simulink model "board_virgin_lab2"  (R2015a)
settings: Solver=ode3  StartTime=0.0  StopTime=inf  FixedStep=0.001  RelTol=1e-3
values from neighbouring files (symbols this model uses):
  T1gain = Pt1(1)    [callback.m]
  T1offset = Pt1(2)    [callback.m]
  T2gain = Pt2(1)    [callback.m]
  T2offset = Pt2(2)    [callback.m]
  Xgain = Px(1)    [callback.m]
  Xoffset = Px(2)    [callback.m]
  Ygain = Py(1)    [callback.m]
  Yoffset = Py(2)    [callback.m]
libraries: PoliArd x14, simulink x4
settings Model: ExtModeTrigDuration=2  Creator=User  LastModifiedBy=user
settings OptimizationCC: OptimizeModelRefInitCode=on  LifeSpan=1
settings DebuggingCC: UnderspecifiedInitializationDetection=Classic  MergeDetectMultiDrivingBlocksExec=none
settings HardwareCC: ProdLargestAtomicInteger=Long  ProdLargestAtomicFloat=Double  ProdEndianess=LittleEndian  ProdHWDeviceType=ARM Compatible->ARM Cortex
settings RTWCC: SystemTargetFile=realtime.tlc  GenerateMakefile=off  TemplateMakefile=realtime.tmf  Description=Run on Target Hardware  RTWVerbose=off
settings ERTTargetCC: CombineOutputUpdateFcns=off  ExtModeTransport=3  ExtModeMexFile=ext_serial_win32_comm_rtt  ExtModeMexArgs=0 1 9600  InlinedParameterPlacement=Hierarchical  ERTSrcFileBannerTemplate=realtime_code_template.cgt  ERTHdrFileBannerTemplate=realtime_code_template.cgt  ERTDataSrcFileTemplate=realtime_code_template.cgt  ERTDataHdrFileTemplate=realtime_code_template.cgt  ERTCustomFileTemplate=realtime_file_process.tlc

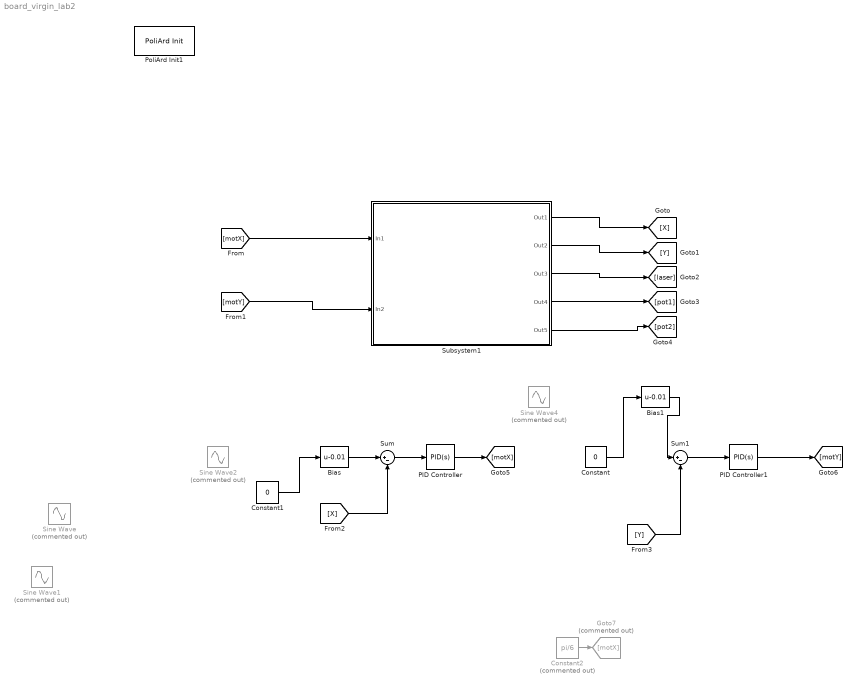
== system board_virgin_lab2 ==
  Bias : Bias  Bias=-0.01
  Bias1 : Bias  Bias=-0.01
  Constant : Constant  Value=0
  Constant1 : Constant  Value=0
  Constant2 : Constant  Commented=on  Value=pi/6
  Goto7 : Goto  Commented=on  GotoTag=motX
  PID Controller : simulink/Continuous/PID Controller  Controller=PID  TimeDomain=Continuous-time  SampleTime=-1  IntegratorMethod=Forward Euler  FilterMethod=Forward Euler  Form=Parallel  UseFilter=on  ControllerParametersSource=internal  P=3  I=1.5  D=2.5  N=5.45  InitialConditionSource=internal  InitialConditionForIntegrator=0  InitialConditionForFilter=0  ExternalReset=none  LimitOutput=off  UpperSaturationLimit=inf  LowerSaturationLimit=-inf  LinearizeAsGain=on  AntiWindupMode=none  Kb=1  TrackingMode=off  Kt=1  PParamMin=[]  PParamMax=[]  IParamMin=[]  IParamMax=[]  DParamMin=[]  DParamMax=[]  NParamMin=[]  NParamMax=[]  KbParamMin=[]  KbParamMax=[]  KtParamMin=[]  KtParamMax=[]  POutMin=[]  POutMax=[]  IOutMin=[]  IOutMax=[]  DOutMin=[]  DOutMax=[]  NOutMin=[]  NOutMax=[]  KbOutMin=[]  KbOutMax=[]  KtOutMin=[]  KtOutMax=[]  IntegratorOutMin=[]  IntegratorOutMax=[]  FilterOutMin=[]  FilterOutMax=[]  SumOutMin=[]  SumOutMax=[]  SumI1OutMin=[]  SumI1OutMax=[]  SumI2OutMin=[]  SumI2OutMax=[]  SumI3OutMin=[]  SumI3OutMax=[]  SumDOutMin=[]  SumDOutMax=[]  SaturationOutMin=[]  SaturationOutMax=[]  IntegratorContinuousStateAttributes=''  IntegratorStateMustResolveToSignalObject=off  IntegratorRTWStateStorageClass=Auto  FilterContinuousStateAttributes=''  FilterStateMustResolveToSignalObject=off  FilterRTWStateStorageClass=Auto  DifferentiatorICPrevScaledInput=0  DifferentiatorOutMin=[]  DifferentiatorOutMax=[]
  PID Controller1 : simulink/Continuous/PID Controller  Controller=PID  TimeDomain=Continuous-time  SampleTime=-1  IntegratorMethod=Forward Euler  FilterMethod=Forward Euler  Form=Parallel  UseFilter=on  ControllerParametersSource=internal  P=3  I=1.5  D=2.5  N=5.45  InitialConditionSource=internal  InitialConditionForIntegrator=0  InitialConditionForFilter=0  ExternalReset=none  LimitOutput=off  UpperSaturationLimit=inf  LowerSaturationLimit=-inf  LinearizeAsGain=on  AntiWindupMode=none  Kb=1  TrackingMode=off  Kt=1  PParamMin=[]  PParamMax=[]  IParamMin=[]  IParamMax=[]  DParamMin=[]  DParamMax=[]  NParamMin=[]  NParamMax=[]  KbParamMin=[]  KbParamMax=[]  KtParamMin=[]  KtParamMax=[]  POutMin=[]  POutMax=[]  IOutMin=[]  IOutMax=[]  DOutMin=[]  DOutMax=[]  NOutMin=[]  NOutMax=[]  KbOutMin=[]  KbOutMax=[]  KtOutMin=[]  KtOutMax=[]  IntegratorOutMin=[]  IntegratorOutMax=[]  FilterOutMin=[]  FilterOutMax=[]  SumOutMin=[]  SumOutMax=[]  SumI1OutMin=[]  SumI1OutMax=[]  SumI2OutMin=[]  SumI2OutMax=[]  SumI3OutMin=[]  SumI3OutMax=[]  SumDOutMin=[]  SumDOutMax=[]  SaturationOutMin=[]  SaturationOutMax=[]  IntegratorContinuousStateAttributes=''  IntegratorStateMustResolveToSignalObject=off  IntegratorRTWStateStorageClass=Auto  FilterContinuousStateAttributes=''  FilterStateMustResolveToSignalObject=off  FilterRTWStateStorageClass=Auto  DifferentiatorICPrevScaledInput=0  DifferentiatorOutMin=[]  DifferentiatorOutMax=[]
  PoliArd Init1 : PoliArd/PoliArd Init
  Sine Wave : Sin  Commented=on  Amplitude=200  Bias=2000  Frequency=2 * 3.14  SampleTime=0
  Sine Wave1 : Sin  Commented=on  Amplitude=200  Bias=2000  Frequency=2 * 3.14  Phase=pi/2  SampleTime=0
  Sine Wave2 : Sin  Commented=on  Amplitude=0.04  Frequency=2*pi*0.25  SampleTime=0
  Sine Wave4 : Sin  Commented=on  Amplitude=0.04  Frequency=2*pi*0.25  Phase=pi/2  SampleTime=0
  Subsystem1 : Subsystem
  Sum : Sum  Inputs=|+-
  Sum1 : Sum  Inputs=|+-
  wires:
  Subsystem1/1(Out1) -> [X]
  Subsystem1/2(Out2) -> [Y]
  Subsystem1/3(Out3) -> [laser]
  Subsystem1/4(Out4) -> [pot1]
  Subsystem1/5(Out5) -> [pot2]
  [motX] -> Subsystem1/1(In1)
  [motY] -> Subsystem1/2(In2)
  [X] -> Sum/2
  Sum/1 -> PID Controller/1
  PID Controller/1 -> [motX]
  PID Controller1/1 -> [motY]
  Sum1/1 -> PID Controller1/1
  [Y] -> Sum1/2
  Constant2/1 -> Goto7/1
  Bias/1 -> Sum/1
  Bias1/1 -> Sum1/1
  Constant/1 -> Bias1/1
  Constant1/1 -> Bias/1

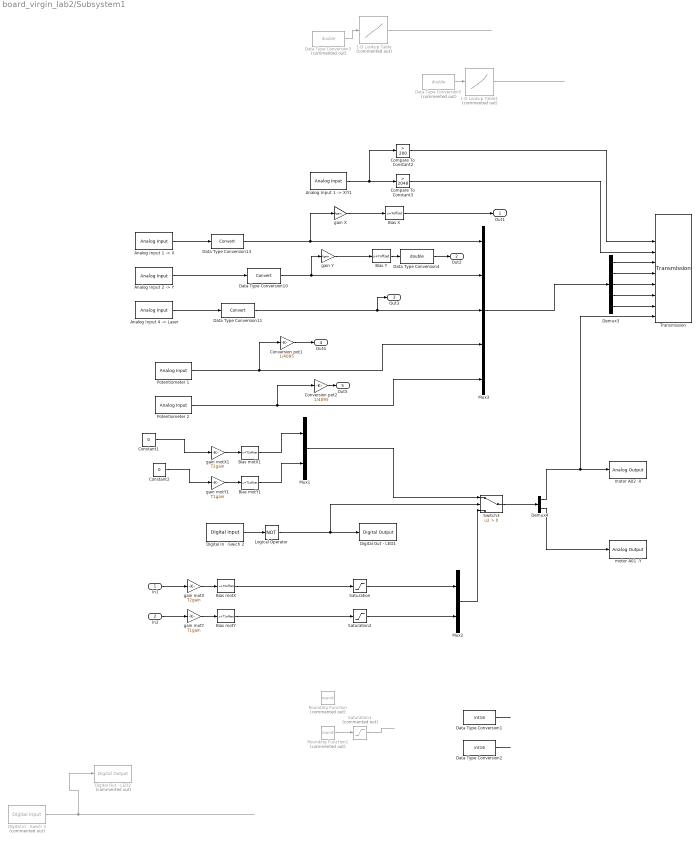
== system board_virgin_lab2/Subsystem1 ==
  In1 : Inport
  In2 : Inport  Port=2
  1-D Lookup Table : Lookup_n-D  Commented=on  NumberOfTableDimensions=1  BreakpointsForDimension1=[870 1250 2036 2836 3410]  Table=-[-127.5 -80 0 80 127.5] * 1e-3  InternalRulePriority=Speed  RndMeth=Simplest  InputSameDT=on
  1-D Lookup Table1 : Lookup_n-D  Commented=on  NumberOfTableDimensions=1  BreakpointsForDimension1=[890 1370 2040 2690 3409]  Table=-[-97.5 -50 0 50 110]*1e-3  InternalRulePriority=Speed  RndMeth=Simplest  InputSameDT=on
  "Analog Input 1 -> X" : PoliArd/Analog Input  AIpin_mask=1  AIsample=-1
  "Analog Input 1 -> X/Y1" : PoliArd/Analog Input  AIpin_mask=7  AIsample=-1
  "Analog Input 2 -> Y" : PoliArd/Analog Input  AIpin_mask=2  AIsample=-1
  "Analog Input 4 -> Laser" : PoliArd/Analog Input  AIpin_mask=4  AIsample=-1
  Bias X : Bias  Bias=Xoffset
  Bias Y : Bias  Bias=Yoffset
  Bias motX : Bias  Bias=T2offset
  Bias motX1 : Bias  Bias=T2offset
  Bias motY : Bias  Bias=T1offset
  Bias motY1 : Bias  Bias=T1offset
  Compare To Constant2 : simulink/Logic and Bit Operations/Compare To Constant  relop=>  const=200  OutDataTypeStr=boolean
  Compare To Constant3 : simulink/Logic and Bit Operations/Compare To Constant  relop=>  const=2048  OutDataTypeStr=boolean
  Constant1 : Constant  Value=0
  Constant2 : Constant  Value=0
  Conversion pot1 : Gain  Gain=1/4095
  Conversion pot2 : Gain  Gain=1/4095
  Data Type Conversion1 : DataTypeConversion  OutDataTypeStr=int16
  Data Type Conversion10 : DataTypeConversion
  Data Type Conversion11 : DataTypeConversion
  Data Type Conversion13 : DataTypeConversion
  Data Type Conversion2 : DataTypeConversion  OutDataTypeStr=int16
  Data Type Conversion3 : DataTypeConversion  Commented=on  OutDataTypeStr=double
  Data Type Conversion4 : DataTypeConversion  OutDataTypeStr=double
  Data Type Conversion5 : DataTypeConversion  Commented=on  OutDataTypeStr=double
  Demux3 : Demux  Outputs=5
  Demux4 : Demux  Outputs=2
  Digital In  -Swich 2 : PoliArd/Digital Input  DI_pin=2  DIsample=-1
  Digital In - Swich 3 : PoliArd/Digital Input  Commented=on  DI_pin=3  DIsample=-1
  Digital Out - LED1 : PoliArd/Digital Output  DO_pin=1
  Digital Out - LED2 : PoliArd/Digital Output  Commented=on  DO_pin=2
  Logical Operator : Logic  Operator=NOT  AllPortsSameDT=off  OutDataTypeStr=boolean
  Mux1 : Mux  Inputs=2
  Mux2 : Mux  Inputs=2
  Mux3 : Mux  Inputs=5
  Potentiometer 1 : PoliArd/Analog Input  AIpin_mask=8  AIsample=-1
  Potentiometer 2 : PoliArd/Analog Input  AIpin_mask=9  AIsample=-1
  Rounding Function : Rounding  Commented=on  Operator=round
  Rounding Function1 : Rounding  Commented=on  Operator=round
  Saturation : Saturate  UpperLimit=4095  LowerLimit=0
  Saturation1 : Saturate  Commented=on  UpperLimit=4095  LowerLimit=0
  Saturation2 : Saturate  UpperLimit=4095  LowerLimit=0
  Switch3 : Switch  Criteria=u2 > Threshold
  Transmission : PoliArd/Transmission  sample_freq=100  sig_to_send=6
  gain X : Gain  Gain=Xgain
  gain Y : Gain  Gain=Ygain
  gain motX : Gain  Gain=T2gain
  gain motX1 : Gain  Gain=T2gain
  gain motY : Gain  Gain=T1gain
  gain motY1 : Gain  Gain=T1gain
  motor A01 -Y : PoliArd/Analog Output  DAC_pin_mask=2
  motor A02 -X : PoliArd/Analog Output  DAC_pin_mask=1
  Out1 : Outport
  Out2 : Outport  Port=2
  Out3 : Outport  Port=3
  Out4 : Outport  Port=4
  Out5 : Outport  Port=5
  wires:
  Switch3/1 -> Demux4/1
  Demux4/2 -> motor A01 -Y/1
  Demux4/1 -> Transmission/10, motor A02 -X/1
  "Analog Input 4 -> Laser"/1 -> Data Type Conversion11/1
  Demux3/3 -> Transmission/7
  Compare To Constant2/1 -> Transmission/3
  Demux3/1 -> Transmission/5
  Demux3/2 -> Transmission/6
  Demux3/5 -> Transmission/9
  "Analog Input 1 -> X/Y1"/1 -> Compare To Constant3/1, Compare To Constant2/1
  Compare To Constant3/1 -> Transmission/4
  Demux3/4 -> Transmission/8
  Mux3/1 -> Demux3/1
  Data Type Conversion11/1 -> Out3/1, Mux3/3
  In1/1 -> gain motX/1
  In2/1 -> gain motY/1
  gain motX/1 -> Bias motX/1
  gain motY/1 -> Bias motY/1
  Mux2/1 -> Switch3/3
  Data Type Conversion13/1 -> gain X/1, Mux3/1
  Data Type Conversion10/1 -> gain Y/1, Mux3/2
  "Analog Input 1 -> X"/1 -> Data Type Conversion13/1
  "Analog Input 2 -> Y"/1 -> Data Type Conversion10/1
  Conversion pot2/1 -> Out5/1
  Potentiometer 2/1 -> Conversion pot2/1, Mux3/5
  Conversion pot1/1 -> Out4/1
  Potentiometer 1/1 -> Conversion pot1/1, Mux3/4
  Rounding Function1/1 -> Saturation1/1
  Saturation1/1 -> ?
  Data Type Conversion1/1 -> ?
  Data Type Conversion2/1 -> ?
  Digital In - Swich 3/1 -> Digital Out - LED2/1
  gain motX1/1 -> Bias motX1/1
  gain motY1/1 -> Bias motY1/1
  Bias motX1/1 -> Mux1/1
  Bias motY1/1 -> Mux1/2
  Constant1/1 -> gain motX1/1
  Constant2/1 -> gain motY1/1
  Mux1/1 -> Switch3/1
  Digital In  -Swich 2/1 -> Logical Operator/1
  Logical Operator/1 -> Switch3/2, Digital Out - LED1/1
  Bias motX/1 -> Saturation/1
  Saturation/1 -> Mux2/1
  Bias motY/1 -> Saturation2/1
  Saturation2/1 -> Mux2/2
  gain X/1 -> Bias X/1
  ? -> ?
  ? -> Data Type Conversion3/1
  1-D Lookup Table/1 -> ?
  Data Type Conversion3/1 -> 1-D Lookup Table/1
  Data Type Conversion5/1 -> 1-D Lookup Table1/1
  1-D Lookup Table1/1 -> ?
  Bias X/1 -> Out1/1
  gain Y/1 -> Bias Y/1
  Bias Y/1 -> Data Type Conversion4/1
  Data Type Conversion4/1 -> Out2/1
